simulink model "Power_Unit_sim"  (R2026a)
settings: Solver=VariableStepAuto
PreLoadFcn:
  | modelPath = get_param(bdroot, 'FileName');
  | if ~isempty(modelPath)
  |     modelDir = fileparts(modelPath);
  |     addpath(modelDir);
  |     addpath(fullfile(modelDir, 'Energy Recovery System'));
  |     addpath(fullfile(modelDir, 'Internal Combustion Engine'));
  | end
InitFcn:
  | common_params_init;
  | ers_params_init;
  | ice_params_init;
undefined symbols (not defined in the file or in its folder): Enable_Bidirectional_Interlock
libraries: SignalEditorBlockLib x1
settings Model: Creator=nixiaofeng  LastModifiedBy=nixiaofeng

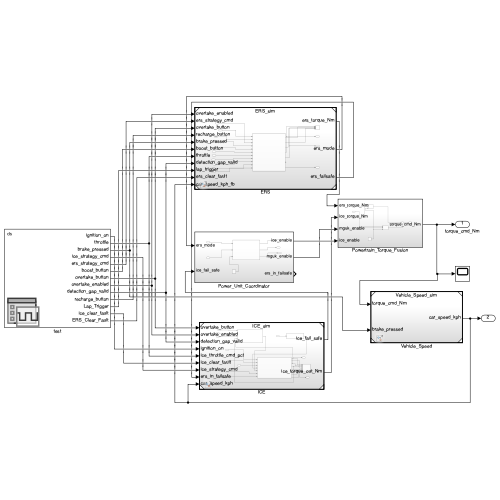
[thumbnail: Simulink's stored preview of the top-level diagram]
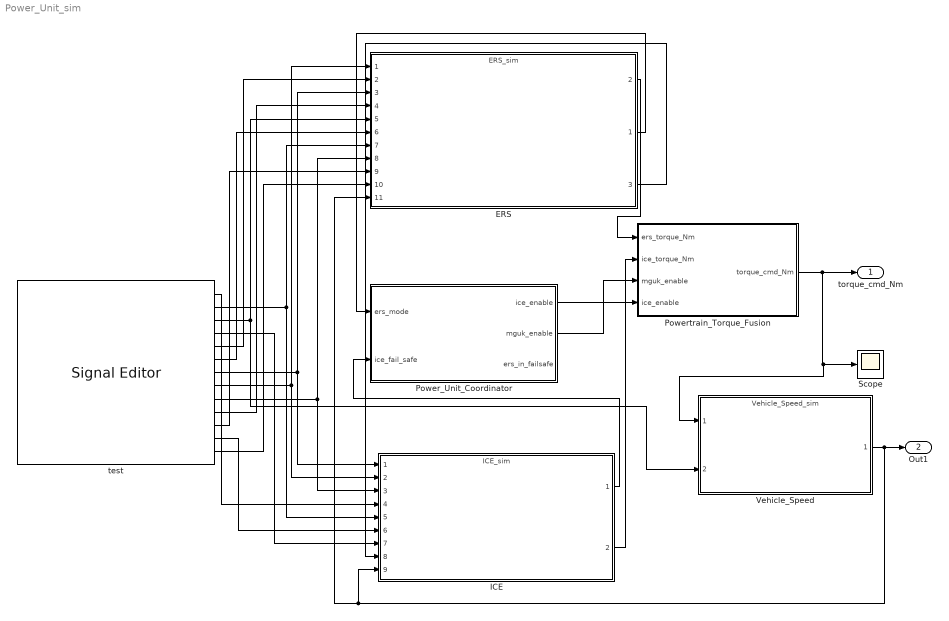
== system Power_Unit_sim ==
  ERS : ModelReference  ModelNameDialog=ERS_sim.slx  SimulationMode=Normal  ModelReferenceVersion=1.87
      settings: PortSchema="{\"entries\":[{\"content\":{\"sides\":[{\"content\":{\"connectorIds\":[\"In1\",\"In2\",\"In3\",\"In4\",\"In5\",\"In6\",\"In7\",\"In8\",\"In9\",\"In10\",\"In11\"]},\"type\":\"ConnectorPlacement.EquallySpacedRectSide\",\"uuid\":\"e3065a4b-2223-41d0-ae8d-97637c2be60c\"},{\"content\":{\"connectorIds\":[\"Out2\",\"Out1\",\"Out3\"],\"side\":\"RIGHT\"},\"type\":\"ConnectorPlacement.EquallySpacedRectSide\",\"uuid\":\"b8900d37-f74b-4a88-b8e3-ceb7d20f8ab0\"},{\"content\":{\"side\":\"TOP\"},\"type\":\"ConnectorPlacement.EquallySpacedRectSide\",\"uuid\":\"ee594b76-c7b7-41d9-b4e3-af6c2a690eb6\"}]},\"type\":\"ConnectorPlacement.EquallySpacedConnector\",\"uuid\":\"e384e75d-6947-4b63-bbd1-ab28cfa37db1\"}],\"packageUris\":[\"http://schema.mathworks.com/mf0/Connector/R2020b\"],\"version\":\"1.0\"}"
  ICE : ModelReference  ModelNameDialog=ICE_sim.slx  SimulationMode=Normal  ModelReferenceVersion=1.26
  Power_Unit_Coordinator : Subsystem
  Powertrain_Torque_Fusion : Subsystem
  Scope : Scope
  Vehicle_Speed : ModelReference  ModelNameDialog=Vehicle_Speed_sim.slx  SimulationMode=Normal  ModelReferenceVersion=1.3
  test : SignalEditorBlockLib/Signal Editor  FileName=/Users/nixiaofeng/Documents/MATLAB/Power Unit/unified_power_unit_test.mat  ActiveScenario=ds  ActiveSignal=ignition_on  IsBus=off  OutputBusObjectStr=Bus: BusObject  SampleTime=0  ZeroCross=off  OutputAfterFinalValue=Setting to zero  Unit=inherit  PreserveSignalName=on  ApplySigPropsToAllScenarios=on  ApplySigPropsToAllSignals=off  SignalPropertySource=Dialog parameters
  torque_cmd_Nm : Outport
  Out1 : Outport  Port=2
  wires:
  Power_Unit_Coordinator/1(ice_enable) -> Powertrain_Torque_Fusion/4(ice_enable)
  Power_Unit_Coordinator/2(mguk_enable) -> Powertrain_Torque_Fusion/3(mguk_enable)
  ERS/1 -> Power_Unit_Coordinator/1(ers_mode)
  ERS/2 -> Powertrain_Torque_Fusion/1(ers_torque_Nm)
  ICE/1 -> Power_Unit_Coordinator/2(ice_fail_safe)
  ICE/2 -> Powertrain_Torque_Fusion/2(ice_torque_Nm)
  Powertrain_Torque_Fusion/1(torque_cmd_Nm) -> Vehicle_Speed/1, Scope/1, torque_cmd_Nm/1
  test/1 -> ICE/4
  test/2 -> ICE/5, ERS/7
  test/3 -> Vehicle_Speed/2, ERS/5
  test/4 -> ICE/7
  test/5 -> ERS/2
  test/6 -> ERS/6
  test/7 -> ICE/1, ERS/3
  test/8 -> ICE/2, ERS/1
  test/9 -> ICE/3, ERS/8
  test/10 -> ERS/4
  test/11 -> ERS/9
  test/12 -> ICE/6
  test/13 -> ERS/10
  Vehicle_Speed/1 -> ICE/9, ERS/11, Out1/1
  ERS/3 -> ICE/8

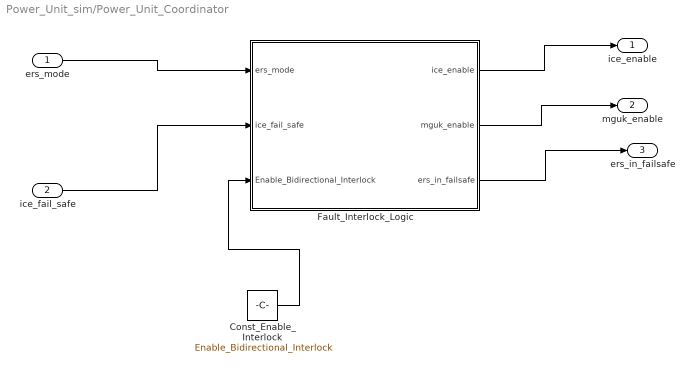
== system Power_Unit_sim/Power_Unit_Coordinator ==
  ers_mode : Inport
  ice_fail_safe : Inport  Port=2
  Const_Enable_Interlock : Constant  Value=Enable_Bidirectional_Interlock
  Fault_Interlock_Logic : MATLAB Function  TreatAsAtomicUnit=on
  ice_enable : Outport
  mguk_enable : Outport  Port=2
  ers_in_failsafe : Outport  Port=3
  wires:
  ers_mode/1 -> Fault_Interlock_Logic/1(ers_mode)
  ice_fail_safe/1 -> Fault_Interlock_Logic/2(ice_fail_safe)
  Const_Enable_Interlock/1 -> Fault_Interlock_Logic/3(Enable_Bidirectional_Interlock)
  Fault_Interlock_Logic/1(ice_enable) -> ice_enable/1
  Fault_Interlock_Logic/2(mguk_enable) -> mguk_enable/1
  Fault_Interlock_Logic/3(ers_in_failsafe) -> ers_in_failsafe/1

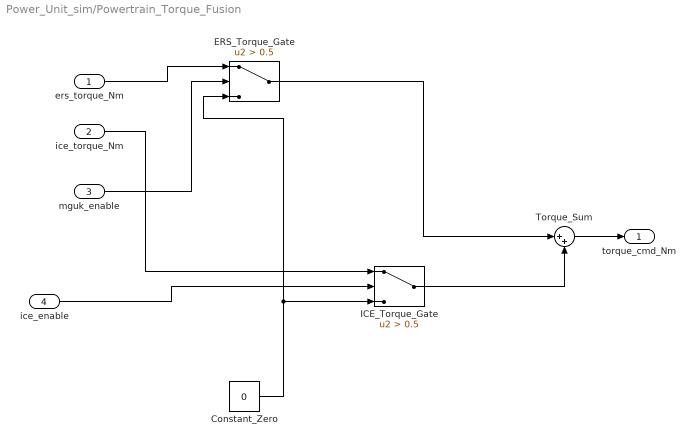
== system Power_Unit_sim/Powertrain_Torque_Fusion ==
  ers_torque_Nm : Inport
  ice_torque_Nm : Inport  Port=2
  mguk_enable : Inport  Port=3
  ice_enable : Inport  Port=4
  Constant_Zero : Constant  Value=0
  ERS_Torque_Gate : Switch  Criteria=u2 > Threshold  Threshold=0.5  SaturateOnIntegerOverflow=off  InputSameDT=off
  ICE_Torque_Gate : Switch  Criteria=u2 > Threshold  Threshold=0.5  SaturateOnIntegerOverflow=off  InputSameDT=off
  Torque_Sum : Sum  Inputs=|++
  torque_cmd_Nm : Outport
  wires:
  ers_torque_Nm/1 -> ERS_Torque_Gate/1
  mguk_enable/1 -> ERS_Torque_Gate/2
  Constant_Zero/1 -> ICE_Torque_Gate/3, ERS_Torque_Gate/3
  ice_enable/1 -> ICE_Torque_Gate/2
  ice_torque_Nm/1 -> ICE_Torque_Gate/1
  Torque_Sum/1 -> torque_cmd_Nm/1
  ERS_Torque_Gate/1 -> Torque_Sum/1
  ICE_Torque_Gate/1 -> Torque_Sum/2

== matlab function Power_Unit_sim/Power_Unit_Coordinator/Fault_Interlock_Logic ==
  data: ers_mode input; ice_enable output; ice_fail_safe input; Enable_Bidirectional_Interlock input; mguk_enable output; ers_in_failsafe output
function [ice_enable, mguk_enable, ers_in_failsafe] = Fault_Interlock_Logic(ers_mode, ice_fail_safe, Enable_Bidirectional_Interlock)
    % 1. 判断 ERS 是否处于 Fail_Safe 状态 (假设模式 3 代表 Fail_Safe)
    ers_in_failsafe = (double(ers_mode) == 3);
    
    % 2. 单向互锁：ERS 故障时切断 ICE 输出
    ice_enable = ~ers_in_failsafe;
    
    % 3. 双向互锁（可选分支）
    if Enable_Bidirectional_Interlock
        mguk_enable = ~ice_fail_safe;   % ICE 故障时反向切断 MGU-K 输出
    else
        mguk_enable = true;             % 默认：ICE 故障不影响 MGU-K
    end
end
